simulink model "exp_4"  (R2020a)
settings: Solver=VariableStepAuto  StartTime=0.0  StopTime=20.0  RelTol=1e-3
settings Model: Creator=hp  LastModifiedBy=hp

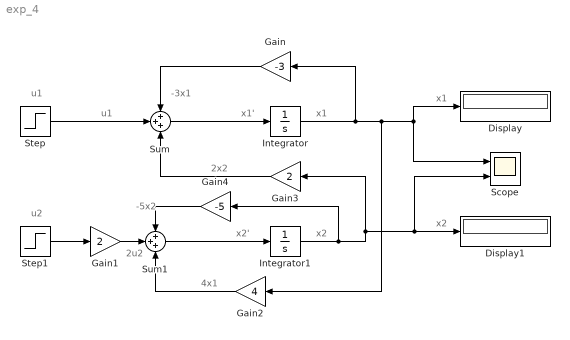
== system exp_4 ==
  note: x2
  note: x2'
  note: -5x2
  note: 2u2
  note: 4x1
  note: u2
  note: u1
  note: u1
  note: -3x1
  note: x1
  note: x1'
  note: 2x2
  note: x1
  note: x2
  Display : Display
  Display1 : Display
  Gain : Gain  Gain=-3
  Gain1 : Gain  Gain=2
  Gain2 : Gain  Gain=4
  Gain3 : Gain  Gain=2
  Gain4 : Gain  Gain=-5
  Integrator : Integrator
  Integrator1 : Integrator
  Scope : Scope  NumInputPorts=2
  Step : Step  Time=0  SampleTime=0
  Step1 : Step  Time=0  SampleTime=0
  Sum : Sum  Inputs=+++
  Sum1 : Sum  Inputs=+++
  wires:
  Sum/1 -> Integrator/1
  Integrator/1 -> Gain/1, Gain2/1, Display/1, Scope/1
  Step/1 -> Sum/2
  Gain/1 -> Sum/1
  Step1/1 -> Gain1/1
  Integrator1/1 -> Gain4/1, Scope/2, Display1/1, Gain3/1
  Gain3/1 -> Sum/3
  Gain2/1 -> Sum1/3
  Gain1/1 -> Sum1/2
  Gain4/1 -> Sum1/1
  Sum1/1 -> Integrator1/1
